simulink model "TOAD_Simulation_2025a"  (R2025a)
settings: Solver=VariableStepAuto  StartTime=0.0  StopTime=60  RelTol=1e-3
InitFcn:
  | LoadTOADSim
values from neighbouring files (symbols this model uses):
  constantsASTRA = 1.275    [Model_Vars.sldd]
  dt = 0.005    [Model_Vars.sldd]
  dt_SIM = 1/500    (= 0.002)    [LoadTOADSim.m]
  IMU_Rate = 500    [LoadTOADSim.m]    (also in Model_Vars.sldd = 1000.0)
  magDistMatrix = [dM_xx, dM_xy, dM_xz ... (first row only)    [LoadTOADSim.m]    (also in Model_Vars.sldd = 1.0 0.0 0.0 0.0 1.0 0.0 0.0 0.0 1.0)
  x0 = [1; zeros(12,1); constants6DoF.OxMass; constants6DoF.FuMass]    [LoadTOADSim.m]    (also in Model_Vars.sldd = 1.0 0.0 0.0 0.0 0.0 0.0 0.0 0.0 0.0 0.0 0.0 0.0 0.0 20.78 19)
undefined symbols (not defined in the file or in its folder): constantsTOAD
libraries: aerolibnav x2, simulink x1
settings Model: DataDictionary=Model_Vars.sldd  SimulationMode=accelerator  PacingRate=5  Creator=antho  LastModifiedBy=alex2

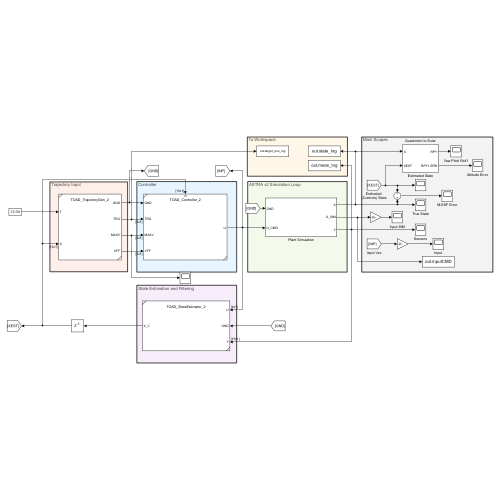
[thumbnail: Simulink's stored preview of the top-level diagram]
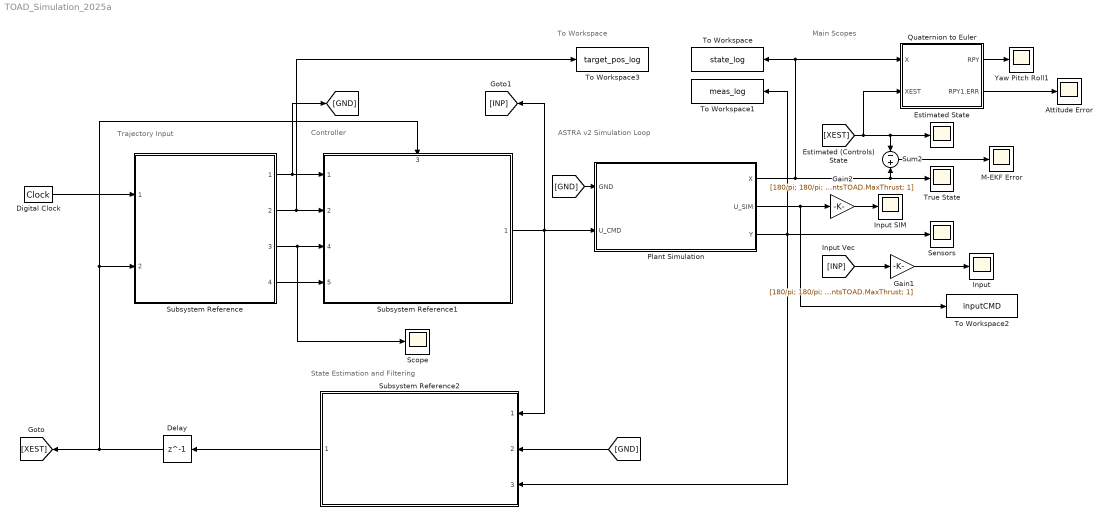
== system TOAD_Simulation_2025a ==
  note: To Workspace
  note: Main Scopes
  note: Trajectory Input
  note: State Estimation and Filtering
  note: Controller
  note: ASTRA v2 Simulation Loop
  Attitude Error : Scope
      settings: ActiveDisplayYMinimum=-3.4509331014700138  ActiveDisplayYMaximum=3.9236687962401184  DataLoggingVariableName=ScopeData9
  Delay : Delay  DelayLength=1  InitialCondition=[1; zeros(14,1)]
  Digital Clock : DigitalClock  SampleTime=dt_SIM
  Estimated State : Scope
      settings: ActiveDisplayYMinimum=-1.6597924359386846  ActiveDisplayYMaximum=1.6422673244276358
  Gain1 : Gain  Gain=[180/pi; 180/pi; 1 / constantsTOAD.MaxThrust; 1]
  Gain2 : Gain  Gain=[180/pi; 180/pi; 1 / constantsTOAD.MaxThrust; 1]
  Input : Scope
      settings: ActiveDisplayYMinimum=-0.094181223962027438  ActiveDisplayYMaximum=1.324748903933564  DataLoggingVariableName=ScopeData6
  Input SIM : Scope
      settings: ActiveDisplayYMinimum=-3.5461841191539949  ActiveDisplayYMaximum=4.4763903999303407  DataLoggingVariableName=ScopeData4
  M-EKF Error : Scope
      settings: ActiveDisplayYMinimum=-0.81415794777034378  ActiveDisplayYMaximum=0.77939335770036378  DataLoggingVariableName=ScopeData2
  Plant Simulation : Subsystem
  Quaternion to Euler : Subsystem
  Scope : Scope
      settings: ActiveDisplayYMinimum=-1  ActiveDisplayYMaximum=1  DataLoggingVariableName=ScopeData7
  Sensors : Scope
      settings: ActiveDisplayYMinimum=-4.1268685590385541  ActiveDisplayYMaximum=5.6741562285888891  DataLoggingVariableName=ScopeData3
  Subsystem Reference : Subsystem  ReferencedSubsystem=TOAD_TrajectoryGen_2
  Subsystem Reference1 : Subsystem  ReferencedSubsystem=TOAD_Controller_2
      settings: PortSchema="{\"entries\":[{\"content\":{\"sides\":[{\"content\":{\"connectorIds\":[\"In1\",\"In2\",\"In4\",\"In5\"]},\"type\":\"ConnectorPlacement.EquallySpacedRectSide\",\"uuid\":\"a3b940ed-534e-42a9-9a71-280d025eee1c\"},{\"content\":{\"connectorIds\":[\"Out1\"],\"side\":\"RIGHT\"},\"type\":\"ConnectorPlacement.EquallySpacedRectSide\",\"uuid\":\"7bc6e323-2b4c-40ac-b214-7c98b845c621\"},{\"content\":{\"connectorIds\":[\"In3\"],\"side\":\"TOP\"},\"type\":\"ConnectorPlacement.EquallySpacedRectSide\",\"uuid\":\"eb0bfab0-68c0-42fd-941a-b96e400ba7cb\"}]},\"type\":\"ConnectorPlacement.EquallySpacedConnector\",\"uuid\":\"b1ebaa4a-87c8-494e-a5ce-deec8c62c7be\"}],\"packageUris\":[\"http://schema.mathworks.com/mf0/Connector/R2020b\"],\"version\":\"1.0\"}"
  Subsystem Reference2 : Subsystem  ReferencedSubsystem=TOAD_StateEstimator_2
  Sum2 : Sum  Inputs=-|+
  To Workspace : ToWorkspace  VariableName=state_log  SaveFormat=Timeseries  SampleTime=-1
  To Workspace1 : ToWorkspace  VariableName=meas_log  SaveFormat=Timeseries  SampleTime=-1
  To Workspace2 : ToWorkspace  VariableName=inputCMD  SaveFormat=Timeseries  SampleTime=-1
  To Workspace3 : ToWorkspace  VariableName=target_pos_log  SaveFormat=Timeseries  SampleTime=-1
  True State : Scope
      settings: ActiveDisplayYMinimum=-13.460760271105533  ActiveDisplayYMaximum=57.064298974553147
  Yaw Pitch Roll1 : Scope
      settings: ActiveDisplayYMinimum=-224.99023889502547  ActiveDisplayYMaximum=224.99733749831469  DataLoggingVariableName=ScopeData5
  wires:
  Digital Clock/1 -> Subsystem Reference/1
  Subsystem Reference2/1 -> Delay/1
  [XEST] -> Estimated State/1, Sum2/1, Quaternion to Euler/2(XEST)
  Sum2/1 -> M-EKF Error/1
  Subsystem Reference1/1 -> Subsystem Reference2/1, [INP], Plant Simulation/2(U_CMD)
  Subsystem Reference/1 -> [GND], Subsystem Reference1/1
  [INP] -> Gain1/1
  Gain1/1 -> Input/1
  Gain2/1 -> Input SIM/1
  Plant Simulation/2(U_SIM) -> To Workspace2/1, Gain2/1
  [GND] -> Subsystem Reference2/2
  Plant Simulation/3(Y) -> Subsystem Reference2/3, Sensors/1, To Workspace1/1
  Plant Simulation/1(X) -> Sum2/2, True State/1, To Workspace/1, Quaternion to Euler/1(X)
  [GND] -> Plant Simulation/1(GND)
  Delay/1 -> Subsystem Reference1/3, Subsystem Reference/2, [XEST]
  Subsystem Reference/2 -> To Workspace3/1, Subsystem Reference1/2
  Quaternion to Euler/1(RPY) -> Yaw Pitch Roll1/1
  Quaternion to Euler/2(RPY1.ERR) -> Attitude Error/1
  Subsystem Reference/3 -> Scope/1, Subsystem Reference1/4
  Subsystem Reference/4 -> Subsystem Reference1/5

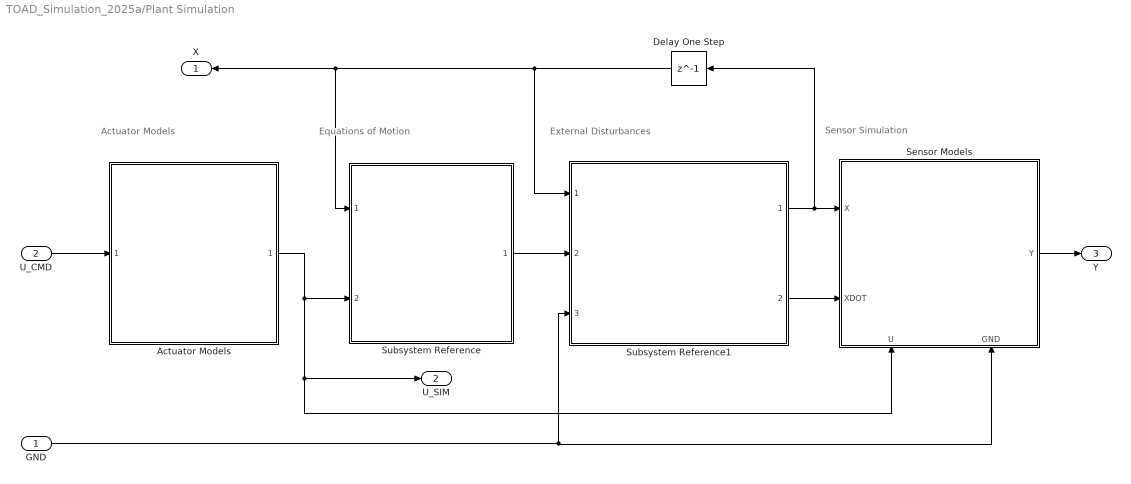
== system TOAD_Simulation_2025a/Plant Simulation ==
  note: Equations of Motion
  note: Actuator Models
  note: External Disturbances
  note: Sensor Simulation
  GND : Inport
  U_CMD : Inport  Port=2
  Actuator Models : Subsystem  ReferencedSubsystem=Actuator_Models_2
  Delay One Step : Delay  DelayLength=1  InitialCondition=x0
  Sensor Models : Subsystem
      settings: PortSchema="{\"entries\":[{\"content\":{\"sides\":[{\"content\":{\"connectorIds\":[\"In1\",\"In2\"]},\"type\":\"ConnectorPlacement.EquallySpacedRectSide\",\"uuid\":\"9bc4a206-bba4-4c50-88a9-89b0392ab722\"},{\"content\":{\"connectorIds\":[\"Out1\"],\"side\":\"RIGHT\"},\"type\":\"ConnectorPlacement.EquallySpacedRectSide\",\"uuid\":\"162bbd17-e1b8-4f29-9191-53e17e38d79d\"},{\"content\":{\"side\":\"TOP\"},\"type\":\"ConnectorPlacement.EquallySpacedRectSide\",\"uuid\":\"c56a23db-6a5c-435f-99fd-d50fc9dbdc94\"},{\"content\":{\"connectorIds\":[\"In3\",\"In4\"],\"side\":\"BOTTOM\"},\"type\":\"ConnectorPlacement.EquallySpacedRectSide\",\"uuid\":\"e0c2a0dc-3b7a-40ac-8345-28e7bf7b9405\"}]},\"type\":\"ConnectorPlacement.EquallySpacedConnector\",\"uuid\":\"d1c29f55-9be5-4f45-9d70-06beba2c2f44\"}],\"packageUris\":[\"http://schema.mathworks.com/mf0/Connector/R2020b\"],\"version\":\"1.0\"}"
  Subsystem Reference : Subsystem  ReferencedSubsystem=Vehicle_Dynamics_2
  Subsystem Reference1 : Subsystem  ReferencedSubsystem=Dist_Models_Integrator_2
  X : Outport
  U_SIM : Outport  Port=2
  Y : Outport  Port=3
  wires:
  Sensor Models/1(Y) -> Y/1
  Subsystem Reference1/1 -> Delay One Step/1, Sensor Models/1(X)
  Subsystem Reference1/2 -> Sensor Models/2(XDOT)
  Actuator Models/1 -> Subsystem Reference/2, U_SIM/1, Sensor Models/3(U)
  Subsystem Reference/1 -> Subsystem Reference1/2
  U_CMD/1 -> Actuator Models/1
  GND/1 -> Subsystem Reference1/3, Sensor Models/4(GND)
  Delay One Step/1 -> Subsystem Reference1/1, Subsystem Reference/1, X/1

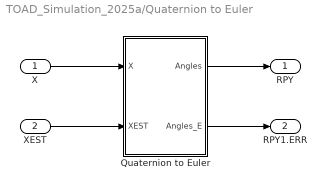
== system TOAD_Simulation_2025a/Quaternion to Euler ==
  X : Inport
  XEST : Inport  Port=2
  Quaternion to Euler : MATLAB Function  TreatAsAtomicUnit=on
  RPY : Outport
  RPY1.ERR : Outport  Port=2
  wires:
  X/1 -> Quaternion to Euler/1(X)
  Quaternion to Euler/1(Angles) -> RPY/1
  XEST/1 -> Quaternion to Euler/2(XEST)
  Quaternion to Euler/2(Angles_E) -> RPY1.ERR/1

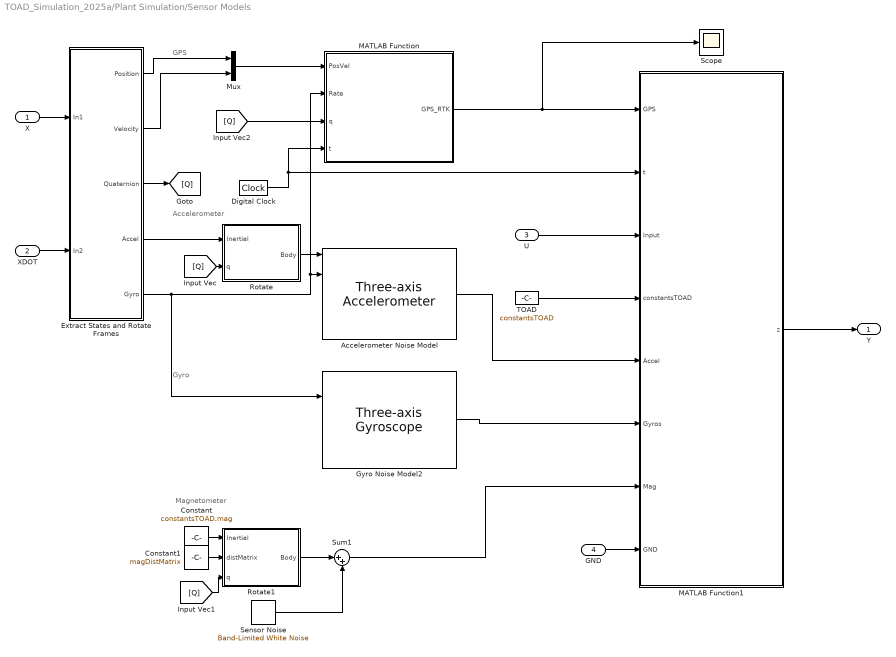
== system TOAD_Simulation_2025a/Plant Simulation/Sensor Models ==
  note: Gyro
  note: Accelerometer
  note: Magnetometer
  note: GPS
  X : Inport  PortDimensions=[15,1]
  XDOT : Inport  Port=2  PortDimensions=[15,1]
  U : Inport  Port=3
  GND : Inport  Port=4
  Accelerometer Noise Model : aerolibnav/Three-axis Accelerometer  units=Metric (MKS)  acc=[0 0 0.15]  gtype=on  dtype_a=on  w_a=190  z_a=0.707  a_sf_cc=eye(3)  a_bias=accelBias  a_Ts=1 / IMU_Rate  a_rand=on  a_seeds=[23093 23094 23095]  a_pow=ones(1,3) * 0.008^2 * 1 / IMU_Rate  a_sat="[-inf  -inf  -inf  inf inf inf]"
  Constant : Constant  Value=constantsTOAD.mag
  Constant1 : Constant  Value=magDistMatrix
  Digital Clock : DigitalClock  SampleTime=dt_SIM
  Extract States and Rotate Frames : Subsystem
  Gyro Noise Model2 : aerolibnav/Three-axis Gyroscope  dtype_g=on  w_g=190  z_g=0.707  g_sf_cc=eye(3)  g_bias=gyroBias  g_sen=0  g_Ts=1 / IMU_Rate  g_rand=on  g_seeds=[23093 23094 23095]  g_pow=ones(1,3) * 0.003^2 * dt  g_sat="[-inf  -inf  -inf  inf inf inf]"
  MATLAB Function : MATLAB Function  TreatAsAtomicUnit=on
  MATLAB Function1 : MATLAB Function  TreatAsAtomicUnit=on
  Mux : Mux  Inputs=2
  Rotate : MATLAB Function  TreatAsAtomicUnit=on
  Rotate1 : MATLAB Function  TreatAsAtomicUnit=on
  Scope : Scope
      settings: ActiveDisplayYMinimum=-1  ActiveDisplayYMaximum=1  DataLoggingVariableName=ScopeData10
  Sensor Noise : simulink/Sources/Band-Limited White Noise  Cov=(4E-4)^2  Ts=dt_SIM  seed=[23341,23342,23343]
  Sum1 : Sum  Inputs=|++
  TOAD : Constant  Value=constantsTOAD  OutDataTypeStr=Bus: slBus1
  Y : Outport
  wires:
  X/1 -> Extract States and Rotate Frames/1(In1)
  XDOT/1 -> Extract States and Rotate Frames/2(In2)
  Digital Clock/1 -> MATLAB Function/4(t), MATLAB Function1/2(t)
  Extract States and Rotate Frames/5(Gyro) -> Accelerometer Noise Model/2, MATLAB Function/2(Rate), Gyro Noise Model2/1
  Extract States and Rotate Frames/3(Quaternion) -> [Q]
  Rotate/1(Body) -> Accelerometer Noise Model/1
  Extract States and Rotate Frames/4(Accel) -> Rotate/1(Inertial)
  [Q] -> Rotate/2(q)
  Constant/1 -> Rotate1/1(Inertial)
  [Q] -> Rotate1/3(q)
  Sensor Noise/1 -> Sum1/2
  Rotate1/1(Body) -> Sum1/1
  Sum1/1 -> MATLAB Function1/7(Mag)
  MATLAB Function/1(GPS_RTK) -> Scope/1, MATLAB Function1/1(GPS)
  Accelerometer Noise Model/1 -> MATLAB Function1/5(Accel)
  Gyro Noise Model2/1 -> MATLAB Function1/6(Gyros)
  MATLAB Function1/1(z) -> Y/1
  TOAD/1 -> MATLAB Function1/4(constantsTOAD)
  Extract States and Rotate Frames/2(Velocity) -> Mux/2
  Mux/1 -> MATLAB Function/1(PosVel)
  Extract States and Rotate Frames/1(Position) -> Mux/1
  U/1 -> MATLAB Function1/3(Input)
  GND/1 -> MATLAB Function1/8(GND)
  Constant1/1 -> Rotate1/2(distMatrix)
  [Q] -> MATLAB Function/3(q)

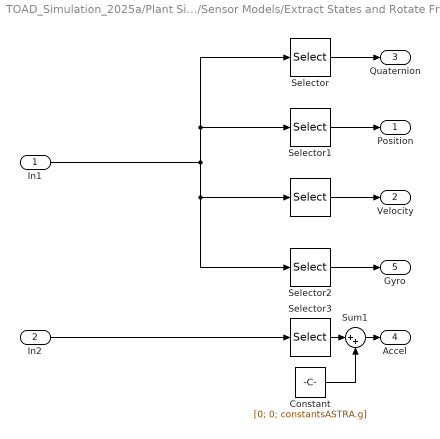
== system TOAD_Simulation_2025a/Plant Simulation/Sensor Models/Extract States and Rotate Frames ==
  In1 : Inport
  In2 : Inport  Port=2
  "  " : Selector  IndexOptions=Index vector (dialog)  Indices=[8:10]  OutputSizes=1
  Constant : Constant  Value=[0; 0; constantsASTRA.g]
  Selector : Selector  IndexOptions=Index vector (dialog)  Indices=[1:4]  OutputSizes=1
  Selector1 : Selector  IndexOptions=Index vector (dialog)  Indices=[5:7]  OutputSizes=1
  Selector2 : Selector  IndexOptions=Index vector (dialog)  Indices=[11:13]  OutputSizes=1
  Selector3 : Selector  IndexOptions=Index vector (dialog)  Indices=[8:10]  OutputSizes=1
  Sum1 : Sum  Inputs=|++
  Position : Outport
  Velocity : Outport  Port=2
  Quaternion : Outport  Port=3
  Accel : Outport  Port=4
  Gyro : Outport  Port=5
  wires:
  Selector/1 -> Quaternion/1
  Selector1/1 -> Position/1
  "  "/1 -> Velocity/1
  Selector2/1 -> Gyro/1
  Selector3/1 -> Sum1/1
  Sum1/1 -> Accel/1
  Constant/1 -> Sum1/2
  In1/1 -> Selector1/1, Selector/1, Selector2/1, "  "/1
  In2/1 -> Selector3/1

== matlab function TOAD_Simulation_2025a/Quaternion to Euler/Quaternion to Euler ==
  data: X input; Angles output; XEST input; Angles_E output
function [Angles, Angles_E] = q2eul(X, XEST)

% Complete quaternion & error quaternion
q = X(1:4);
qest = XEST(1:4);

Q_Conj = [qest(1); -qest(2:4)];
qerr = HamiltonianProd(Q_Conj) * q;
if qerr(1) < 0
    qerr = -qerr;
end

% Quaternion to Euler Angles
Roll = atan2(2*(q(1) * q(2) + q(3) * q(4)), 1 - 2*(q(2)^2 + q(3)^2));
Pitch = asin(2*(q(1) * q(3) - q(4) * q(2)));
Yaw = atan2(2*(q(1) * q(4) + q(2) * q(3)), 1 - 2*(q(3)^2 + q(4)^2));

% Error Euler Angles
Roll_E = atan2(2*(qerr(1) * qerr(2) + qerr(3) * qerr(4)), 1 - 2*(qerr(2)^2 + qerr(3)^2));
Pitch_E = asin(2*(qerr(1) * qerr(3) - qerr(4) * qerr(2)));
Yaw_E = atan2(2*(qerr(1) * qerr(4) + qerr(2) * qerr(3)), 1 - 2*(qerr(3)^2 + qerr(4)^2));


% Angle Vector
Angles = [Roll; Pitch; Yaw] * 180/pi;
Angles_E = [Roll_E; Pitch_E; Yaw_E] * 180/pi;

== matlab function TOAD_Simulation_2025a/Plant Simulation/Sensor Models/Rotate ==
  data: Inertial input; Body output; q input
function Body = Rotate(Inertial, q)
Body = quatRot(q) * Inertial;

== matlab function TOAD_Simulation_2025a/Plant Simulation/Sensor Models/Rotate1 ==
  data: Inertial input; distMatrix input; Body output; q input
function Body = Rotate(Inertial, distMatrix, q)
Body = quatRot(q) * (distMatrix * Inertial + 0.05 * ones(3,1));

== matlab function TOAD_Simulation_2025a/Plant Simulation/Sensor Models/MATLAB Function ==
  data: PosVel input; Rate input; q input; GPS_RTK output; t input
function GPS_RTK = GPS(PosVel, Rate, q, t)

R_b2i = quatRot(q)';
GPS_RTK = GPS_Sim(PosVel, Rate, R_b2i, t);

== matlab function TOAD_Simulation_2025a/Plant Simulation/Sensor Models/MATLAB Function1 ==
  settings: updateMethod=DISCRETE
  data: GPS input; t input; Input input; constantsTOAD input; Accel input; z output; Gyros input; Mag input; GND input
function z = SensorFrequency(GPS, t, Input, constantsTOAD, Accel, Gyros, Mag, GND)
%% Add Thrust Varying Oscillation
persistent phase lastT
if isempty(phase)
    phase = 0;
    lastT = 0;
end
dt = t - lastT;
lastT = t;

% Thrust vibration generator
Track = [1.3525    42.6278];
THRUST = 0; %Input(3) / constantsTOAD.MaxThrust * 100;
w = 2 * pi * (Track(1) * THRUST + Track(2) + 1 * randn());
phase = phase + w * dt;
MaxAmplAccel = 7;
MaxAmplGyro = 0.2;
Accel = Accel + MaxAmplAccel * THRUST / 100 * sin(phase) * (1 - GND);
Gyros = Gyros + MaxAmplGyro * THRUST / 100 * sin(phase) * (1 - GND);
z = [Accel; Gyros; Mag; GPS];
